simulink model "QD2_MissionCtrl_Swarm_6x_R2021a"  (R2021a)
settings: Solver=ode2  StartTime=0.0  StopTime=inf  FixedStep=0.001  RelTol=1e-3  EnableMultiTasking=on
undefined symbols (not defined in the file): datetime, Host, localhost, m, qc_get_step_size, saved_data
libraries: quarc_library x64, simulink x18, simulink_extras x1
(part 1 of 3)
settings Model: SimulationMode=external  ExtModeTrigDuration=10000  Creator=Admin  LastModifiedBy=jpineros
settings SolverCC: AlgebraicLoopSolver=TrustRegion  PositivePriorityOrder=on
settings DataIOCC: ReturnWorkspaceOutputs=off
settings DebuggingCC: SFUnexpectedBacktrackingDiag=warning  SFNoUnconditionalDefaultTransitionDiag=warning  SFExecutionAtInitializationDiag=none  ArithmeticOperatorsInVariantConditions=warning
settings SFSimCC: SimUseLocalCustomCode=off  CustomCodeUndefinedFunction=UseInterfaceOnly
settings RTWCC: Description=QUARC Win64 Target Using Toolchain  SystemTargetFile=quarc_win64.tlc  TemplateMakefile=quarc_default_tmf  RTWUseLocalCustomCode=off  Toolchain=QUARC win64 | nmake (64-bit Windows)  BuildConfiguration=Faster Runs  DLArmComputeVersion=20.02.1
settings CodeAppCC: StateflowObjectComments=on
settings STFCustomTargetCC: ConcurrentExecutionCompliant=on  SystemTargetFile=quarc_win64.tlc
settings GRTTargetCC: TargetLangStandard=C89/C90 (ANSI)  ParMdlRefBuildCompliant=off  CompOptLevelCompliant=off  CombineOutputUpdateFcns=off  MatFileLogging=off  CPPClassGenCompliant=off  GRTInterface=on  ExtMode=on  ExtModeMexFile=quarc_comm  ExtModeMexArgs='-w -d %d -uri %u -URI_Host_V1 tcpip://localhost:18001 -URI_Host_V2 tcpip://localhost:18002 -URI_Host_V3 tcpip://localhost:18003 -URI_Host_V4 tcpip://localhost:18004 -URI_Host_V5 tcpip://localhost:18005 -URI_Host_V6 tcpip://localhost:18006'
settings ConfigComp: CovMetricSettings=dw  CovSaveCumulativeToWorkspaceVar=on  CovSaveSingleToWorkspaceVar=on  CovExternalEMLEnable=off

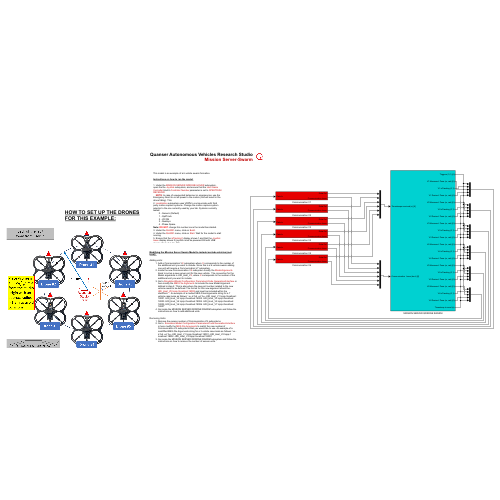
[thumbnail: Simulink's stored preview of the top-level diagram]
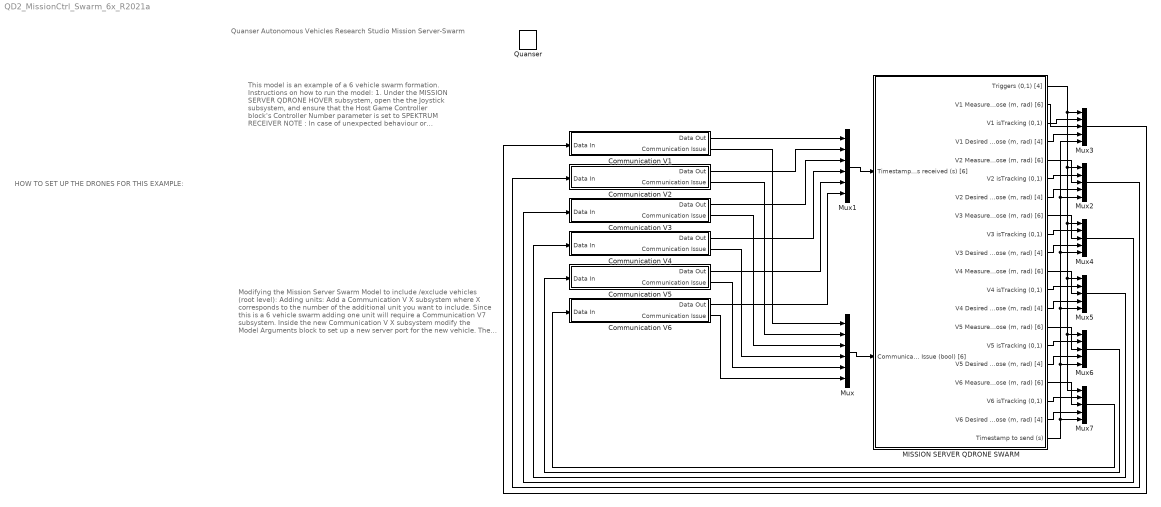
== system QD2_MissionCtrl_Swarm_6x_R2021a ==
  note: Modifying the Mission Server Swarm Model to include /exclude vehicles (root level):
      |
      | Adding units:
      | Add a Communication V X subsystem where X corresponds to the number of the additional unit you want to include. Since this is a 6 vehicle swarm adding one unit will require a Communication V7 subsystem.
      | Inside the new Communication V X subsystem modify the Model Arguments block to set up a new server port for the new vehicle. The convention for the Model arguments is URI_Host_V X , where X corresponds to the number of the additional unit you want to include.
      | Go to Simulation\Model Configuration Parameters\Code Generation\Interface in here modify the MEX-File Arguments to include the new Model Argument defined in step 2. This is also where the new port number related to the new vehicle needs to be defined. The format for this new argument should be -URI_Host_VX tcpip://localhost:1800X and must be included within the identifiers ' ' . An example of a modied MEX-Files Arguments string for a 7 vehicle case looks as follows: '-w -d %d -uri %u -URI_Host_V1 tcpip://localhost:18001 -URI_Host_V2 tcpip://localhost:18002 -URI_Host_V3 tcpip://localhost:18003 -URI_Host_V4 tcpip://localhost:18004 -URI_Host_V5 tcpip://localhost:18005 -URI_Host_V6 tcpip://localhost:18006 -URI_Host_V7 tcpip://localhost:18007'
      | Go inside the MISSION SERVER QDRONE SWARM subsystem and follow the instructions on how to add additional units.
      |
      | Removing Units:
      | Remove the excess number of Communication VX subsystems.
      | Go to Simulation\Model Configuration Parameters\Code Generation\Interface in here modify the MEX-File Arguments to match the new number of Communication VX subsystems that you would like to use. An example of a modifified MEX-File Arguments string for a 3 vehicle case looks as follows: '-w -d %d -uri %u -URI_Host_V1 tcpip://localhost:18001 -URI_Host_V2 tcpip://localhost:18002 -URI_Host_V3 tcpip://localhost:18003'
      | Go inside the MISSION SERVER QDRONE SWARM subsystem and follow the instructions on how to remove the number of excess units.
  note: This model is an example of a 6 vehicle swarm formation.
      |
      | Instructions on how to run the model:
      |
      | 1. Under the MISSION SERVER QDRONE HOVER subsystem, open the the Joystick subsystem, and ensure that the Host Game Controller block's Controller Number parameter is set to SPEKTRUM RECEIVER
      | NOTE : In case of unexpected behaviour or emergencies, use the Emergency Abort to cut all power to the motors (this will result in the drone falling). This
      | 2. Localization subsystem uses VRPN to communicate with third party motion capture systems. Change the motion capture system selector to the one currently used by your lab. Systems currently tested:
      | 0 - Generic (Default)
      | 1 - OptiTrack
      | 2 - VICON
      | 3 - Qualisys
      | 4 - Phase Space
      | Note: DO NOT change this number once the model has started.
      | 3. Under the QUARC menu, click on Build .
      | 4. Under the QUARC menu, click on Start . Wait for the model to start running.
      | 5. Ensure that the isTracking? display shows 1 and that the Joystick Issue display shows 0 (joystick must be powered ON with USB dongle attached to the PC).
      |
      | NOTE : At the start of the model the Comm Issue with Commander display SHOULD display 0. Once the Commander_Stabilizer has successfully connected to the mission server the communication issue flag will update. Landing the QDrones will stop the Commander_Stabilizer model at which point the Comm Issue with Commander should show 1. To close the warning window please stop the Mission_Server_Swarm model.
  note: Quanser Autonomous Vehicles Research Studio
      | Mission Server-Swarm
  note: HOW TO SET UP THE DRONES FOR THIS EXAMPLE:
  Communication V1 : Subsystem
  Communication V2 : Subsystem
  Communication V3 : Subsystem
  Communication V4 : Subsystem
  Communication V5 : Subsystem
  Communication V6 : Subsystem
  MISSION SERVER QDRONE SWARM : Subsystem
  Mux : Mux  Inputs=6
  Mux1 : Mux  Inputs=6
  Mux{2..7} (6 alike) : Mux  Inputs=5
  Quanser : quarc_library/Logos/Quanser
  wires:
  Mux/1 -> MISSION SERVER QDRONE SWARM/2(Communication Issue (bool) [6])
  Mux1/1 -> MISSION SERVER QDRONE SWARM/1(Timestamps received (s) [6])
  MISSION SERVER QDRONE SWARM/3(V1 isTracking (0,1)) -> Mux3/2
  MISSION SERVER QDRONE SWARM/6(V2 isTracking (0,1)) -> Mux2/2
  MISSION SERVER QDRONE SWARM/9(V3 isTracking (0,1)) -> Mux4/2
  MISSION SERVER QDRONE SWARM/12(V4 isTracking (0,1)) -> Mux5/2
  MISSION SERVER QDRONE SWARM/15(V5 isTracking (0,1)) -> Mux6/2
  MISSION SERVER QDRONE SWARM/18(V6 isTracking (0,1)) -> Mux7/2
  MISSION SERVER QDRONE SWARM/1(Triggers (0,1) [4]) -> Mux3/1, Mux2/1, Mux4/1, Mux5/1, Mux6/1, Mux7/1
  MISSION SERVER QDRONE SWARM/4("V1 Desired Pose (m, rad) [4]") -> Mux3/4
  MISSION SERVER QDRONE SWARM/7("V2 Desired Pose (m, rad) [4]") -> Mux2/4
  MISSION SERVER QDRONE SWARM/10("V3 Desired Pose (m, rad) [4]") -> Mux4/4
  MISSION SERVER QDRONE SWARM/13("V4 Desired Pose (m, rad) [4]") -> Mux5/4
  MISSION SERVER QDRONE SWARM/16("V5 Desired Pose (m, rad) [4]") -> Mux6/4
  MISSION SERVER QDRONE SWARM/19("V6 Desired Pose (m, rad) [4]") -> Mux7/4
  MISSION SERVER QDRONE SWARM/20(Timestamp to send (s)) -> Mux3/5, Mux2/5, Mux4/5, Mux5/5, Mux6/5, Mux7/5
  Mux3/1 -> Communication V1/1(Data In)
  Mux2/1 -> Communication V2/1(Data In)
  Mux4/1 -> Communication V3/1(Data In)
  Mux5/1 -> Communication V4/1(Data In)
  Mux6/1 -> Communication V5/1(Data In)
  Mux7/1 -> Communication V6/1(Data In)
  MISSION SERVER QDRONE SWARM/17("V6 Measured Pose (m, rad) [6]") -> Mux7/3
  MISSION SERVER QDRONE SWARM/14("V5 Measured Pose (m, rad) [6]") -> Mux6/3
  MISSION SERVER QDRONE SWARM/11("V4 Measured Pose (m, rad) [6]") -> Mux5/3
  MISSION SERVER QDRONE SWARM/8("V3 Measured  Pose (m, rad) [6]") -> Mux4/3
  MISSION SERVER QDRONE SWARM/5("V2 Measured Pose (m, rad) [6]") -> Mux2/3
  MISSION SERVER QDRONE SWARM/2("V1 Measured Pose (m, rad) [6]") -> Mux3/3
  Communication V1/1(Data Out) -> Mux1/1
  Communication V2/1(Data Out) -> Mux1/2
  Communication V3/1(Data Out) -> Mux1/3
  Communication V4/1(Data Out) -> Mux1/4
  Communication V5/1(Data Out) -> Mux1/5
  Communication V6/1(Data Out) -> Mux1/6
  Communication V1/2(Communication Issue) -> Mux/1
  Communication V2/2(Communication Issue) -> Mux/2
  Communication V3/2(Communication Issue) -> Mux/3
  Communication V4/2(Communication Issue) -> Mux/4
  Communication V5/2(Communication Issue) -> Mux/5
  Communication V6/2(Communication Issue) -> Mux/6

== system QD2_MissionCtrl_Swarm_6x_R2021a/Communication V1 ==
  Data In : Inport
  Constant : Constant
  Detect Communication loss : Subsystem
  Model Argument : quarc_library/Sources/Signals/Model Argument  argument_name=URI_Host_V1  has_value=on  data_type_mode=Specify via dialog  data_type=char  max_length=80  default_value=0  default_string=tcpip://localhost:18001  variable_size=off
      settings: AttributesFormatString=(-%<argument_name>)  SourceProductName=QUARC Targets
  Stream Server : quarc_library/Communications/Basic/Stream Server  uri_source=External input port  uri=tcpip://localhost:18877  send_buffer_size=1460  receive_buffer_size=1460  byte_order=little endian (Intel - LSB first)  optimization=Minimum latency  send_options=Send most recent data  receive_options=Receive most recent data  default_value=zeros(1,1)  sample_time=qc_get_step_size  active=off  implementation=Use blocking I/O in a separate thread  send_fifo_size=1000  receive_fifo_size=1000  send_priority=0  receive_priority=0  send_dimensions=off  receive_dimensions=off  max_dimensions=-1  data_type=Inherited via back propagation  type_expr=BusObject
  "String Display " : quarc_library/Strings/String Display  alignment=center  display_mode=Single line  sample_time=-1  use_new=off
      settings: SourceProductName=QUARC Targets
  Terminator1 : Terminator
  Terminator2 : Terminator
  Data Out : Outport  VectorParamsAs1DForOutWhenUnconnected=off
  Communication Issue : Outport  Port=2  VectorParamsAs1DForOutWhenUnconnected=off
  wires:
  Detect Communication loss/1(Communication Issue (0,1)) -> Communication Issue/1
  Stream Server/1 -> Detect Communication loss/1(State)
  Stream Server/2 -> Detect Communication loss/2(Error)
  Stream Server/4 -> Data Out/1
  Model Argument/1 -> Stream Server/3, "String Display "/1
  Stream Server/5 -> Terminator1/1
  Stream Server/3 -> Terminator2/1
  Data In/1 -> Stream Server/1
  Constant/1 -> Stream Server/2

== system QD2_MissionCtrl_Swarm_6x_R2021a/Communication V2 ==
  Data In : Inport
  Constant : Constant
  Detect Communication loss : Subsystem
  Model Argument : quarc_library/Sources/Signals/Model Argument  argument_name=URI_Host_V2  has_value=on  data_type_mode=Specify via dialog  data_type=char  max_length=80  default_value=0  default_string=tcpip://localhost:18002  variable_size=off
      settings: AttributesFormatString=(-%<argument_name>)  SourceProductName=QUARC Targets
  Stream Server : quarc_library/Communications/Basic/Stream Server  uri_source=External input port  uri=tcpip://localhost:18877  send_buffer_size=1460  receive_buffer_size=1460  byte_order=little endian (Intel - LSB first)  optimization=Minimum latency  send_options=Send most recent data  receive_options=Receive most recent data  default_value=zeros(1,1)  sample_time=qc_get_step_size  active=off  implementation=Use blocking I/O in a separate thread  send_fifo_size=1000  receive_fifo_size=1000  send_priority=0  receive_priority=0  send_dimensions=off  receive_dimensions=off  max_dimensions=-1  data_type=Inherited via back propagation  type_expr=BusObject
  "String Display " : quarc_library/Strings/String Display  alignment=center  display_mode=Single line  sample_time=-1  use_new=off
      settings: SourceProductName=QUARC Targets
  Terminator1 : Terminator
  Terminator2 : Terminator
  Data Out : Outport  VectorParamsAs1DForOutWhenUnconnected=off
  Communication Issue : Outport  Port=2  VectorParamsAs1DForOutWhenUnconnected=off
  wires:
  Constant/1 -> Stream Server/2
  Data In/1 -> Stream Server/1
  Stream Server/3 -> Terminator2/1
  Stream Server/5 -> Terminator1/1
  Model Argument/1 -> "String Display "/1, Stream Server/3
  Stream Server/4 -> Data Out/1
  Stream Server/2 -> Detect Communication loss/2(Error)
  Stream Server/1 -> Detect Communication loss/1(State)
  Detect Communication loss/1(Communication Issue (0,1)) -> Communication Issue/1

== system QD2_MissionCtrl_Swarm_6x_R2021a/Communication V3 ==
  Data In : Inport
  Constant : Constant
  Detect Communication loss : Subsystem
  Model Argument : quarc_library/Sources/Signals/Model Argument  argument_name=URI_Host_V3  has_value=on  data_type_mode=Specify via dialog  data_type=char  max_length=80  default_value=0  default_string=tcpip://localhost:18003  variable_size=off
      settings: AttributesFormatString=(-%<argument_name>)  SourceProductName=QUARC Targets
  Stream Server : quarc_library/Communications/Basic/Stream Server  uri_source=External input port  uri=tcpip://localhost:18877  send_buffer_size=1460  receive_buffer_size=1460  byte_order=little endian (Intel - LSB first)  optimization=Minimum latency  send_options=Send most recent data  receive_options=Receive most recent data  default_value=zeros(1,1)  sample_time=qc_get_step_size  active=off  implementation=Use blocking I/O in a separate thread  send_fifo_size=1000  receive_fifo_size=1000  send_priority=0  receive_priority=0  send_dimensions=off  receive_dimensions=off  max_dimensions=-1  data_type=Inherited via back propagation  type_expr=BusObject
  "String Display " : quarc_library/Strings/String Display  alignment=center  display_mode=Single line  sample_time=-1  use_new=off
      settings: SourceProductName=QUARC Targets
  Terminator1 : Terminator
  Terminator2 : Terminator
  Data Out : Outport  VectorParamsAs1DForOutWhenUnconnected=off
  Communication Issue : Outport  Port=2  VectorParamsAs1DForOutWhenUnconnected=off
  wires:
  Detect Communication loss/1(Communication Issue (0,1)) -> Communication Issue/1
  Stream Server/1 -> Detect Communication loss/1(State)
  Stream Server/2 -> Detect Communication loss/2(Error)
  Stream Server/4 -> Data Out/1
  Model Argument/1 -> Stream Server/3, "String Display "/1
  Stream Server/5 -> Terminator1/1
  Stream Server/3 -> Terminator2/1
  Data In/1 -> Stream Server/1
  Constant/1 -> Stream Server/2

== system QD2_MissionCtrl_Swarm_6x_R2021a/Communication V4 ==
  Data In : Inport
  Constant : Constant
  Detect Communication loss : Subsystem
  Model Argument : quarc_library/Sources/Signals/Model Argument  argument_name=URI_Host_V4  has_value=on  data_type_mode=Specify via dialog  data_type=char  max_length=80  default_value=0  default_string=tcpip://localhost:18004  variable_size=off
      settings: AttributesFormatString=(-%<argument_name>)  SourceProductName=QUARC Targets
  Stream Server : quarc_library/Communications/Basic/Stream Server  uri_source=External input port  uri=tcpip://localhost:18877  send_buffer_size=1460  receive_buffer_size=1460  byte_order=little endian (Intel - LSB first)  optimization=Minimum latency  send_options=Send most recent data  receive_options=Receive most recent data  default_value=zeros(1,1)  sample_time=qc_get_step_size  active=off  implementation=Use blocking I/O in a separate thread  send_fifo_size=1000  receive_fifo_size=1000  send_priority=0  receive_priority=0  send_dimensions=off  receive_dimensions=off  max_dimensions=-1  data_type=Inherited via back propagation  type_expr=BusObject
  "String Display " : quarc_library/Strings/String Display  alignment=center  display_mode=Single line  sample_time=-1  use_new=off
      settings: SourceProductName=QUARC Targets
  Terminator1 : Terminator
  Terminator2 : Terminator
  Data Out : Outport  VectorParamsAs1DForOutWhenUnconnected=off
  Communication Issue : Outport  Port=2  VectorParamsAs1DForOutWhenUnconnected=off
  wires:
  Constant/1 -> Stream Server/2
  Data In/1 -> Stream Server/1
  Stream Server/3 -> Terminator2/1
  Stream Server/5 -> Terminator1/1
  Model Argument/1 -> "String Display "/1, Stream Server/3
  Stream Server/4 -> Data Out/1
  Stream Server/2 -> Detect Communication loss/2(Error)
  Stream Server/1 -> Detect Communication loss/1(State)
  Detect Communication loss/1(Communication Issue (0,1)) -> Communication Issue/1

== system QD2_MissionCtrl_Swarm_6x_R2021a/Communication V5 ==
  Data In : Inport
  Constant : Constant
  Detect Communication loss : Subsystem
  Model Argument : quarc_library/Sources/Signals/Model Argument  argument_name=URI_Host_V5  has_value=on  data_type_mode=Specify via dialog  data_type=char  max_length=80  default_value=0  default_string=tcpip://localhost:18005  variable_size=off
      settings: AttributesFormatString=(-%<argument_name>)  SourceProductName=QUARC Targets
  Stream Server : quarc_library/Communications/Basic/Stream Server  uri_source=External input port  uri=tcpip://localhost:18877  send_buffer_size=1460  receive_buffer_size=1460  byte_order=little endian (Intel - LSB first)  optimization=Minimum latency  send_options=Send most recent data  receive_options=Receive most recent data  default_value=zeros(1,1)  sample_time=qc_get_step_size  active=off  implementation=Use blocking I/O in a separate thread  send_fifo_size=1000  receive_fifo_size=1000  send_priority=0  receive_priority=0  send_dimensions=off  receive_dimensions=off  max_dimensions=-1  data_type=Inherited via back propagation  type_expr=BusObject
  "String Display " : quarc_library/Strings/String Display  alignment=center  display_mode=Single line  sample_time=-1  use_new=off
      settings: SourceProductName=QUARC Targets
  Terminator1 : Terminator
  Terminator2 : Terminator
  Data Out : Outport  VectorParamsAs1DForOutWhenUnconnected=off
  Communication Issue : Outport  Port=2  VectorParamsAs1DForOutWhenUnconnected=off
  wires:
  Detect Communication loss/1(Communication Issue (0,1)) -> Communication Issue/1
  Stream Server/1 -> Detect Communication loss/1(State)
  Stream Server/2 -> Detect Communication loss/2(Error)
  Stream Server/4 -> Data Out/1
  Model Argument/1 -> Stream Server/3, "String Display "/1
  Stream Server/5 -> Terminator1/1
  Stream Server/3 -> Terminator2/1
  Data In/1 -> Stream Server/1
  Constant/1 -> Stream Server/2

== system QD2_MissionCtrl_Swarm_6x_R2021a/Communication V6 ==
  Data In : Inport
  Constant : Constant
  Detect Communication loss : Subsystem
  Model Argument : quarc_library/Sources/Signals/Model Argument  argument_name=URI_Host_V6  has_value=on  data_type_mode=Specify via dialog  data_type=char  max_length=80  default_value=0  default_string=tcpip://localhost:18006  variable_size=off
      settings: AttributesFormatString=(-%<argument_name>)  SourceProductName=QUARC Targets
  Stream Server : quarc_library/Communications/Basic/Stream Server  uri_source=External input port  uri=tcpip://localhost:18877  send_buffer_size=1460  receive_buffer_size=1460  byte_order=little endian (Intel - LSB first)  optimization=Minimum latency  send_options=Send most recent data  receive_options=Receive most recent data  default_value=zeros(1,1)  sample_time=qc_get_step_size  active=off  implementation=Use blocking I/O in a separate thread  send_fifo_size=1000  receive_fifo_size=1000  send_priority=0  receive_priority=0  send_dimensions=off  receive_dimensions=off  max_dimensions=-1  data_type=Inherited via back propagation  type_expr=BusObject
  "String Display " : quarc_library/Strings/String Display  alignment=center  display_mode=Single line  sample_time=-1  use_new=off
      settings: SourceProductName=QUARC Targets
  Terminator1 : Terminator
  Terminator2 : Terminator
  Data Out : Outport  VectorParamsAs1DForOutWhenUnconnected=off
  Communication Issue : Outport  Port=2  VectorParamsAs1DForOutWhenUnconnected=off
  wires:
  Constant/1 -> Stream Server/2
  Data In/1 -> Stream Server/1
  Stream Server/3 -> Terminator2/1
  Stream Server/5 -> Terminator1/1
  Model Argument/1 -> "String Display "/1, Stream Server/3
  Stream Server/4 -> Data Out/1
  Stream Server/2 -> Detect Communication loss/2(Error)
  Stream Server/1 -> Detect Communication loss/1(State)
  Detect Communication loss/1(Communication Issue (0,1)) -> Communication Issue/1

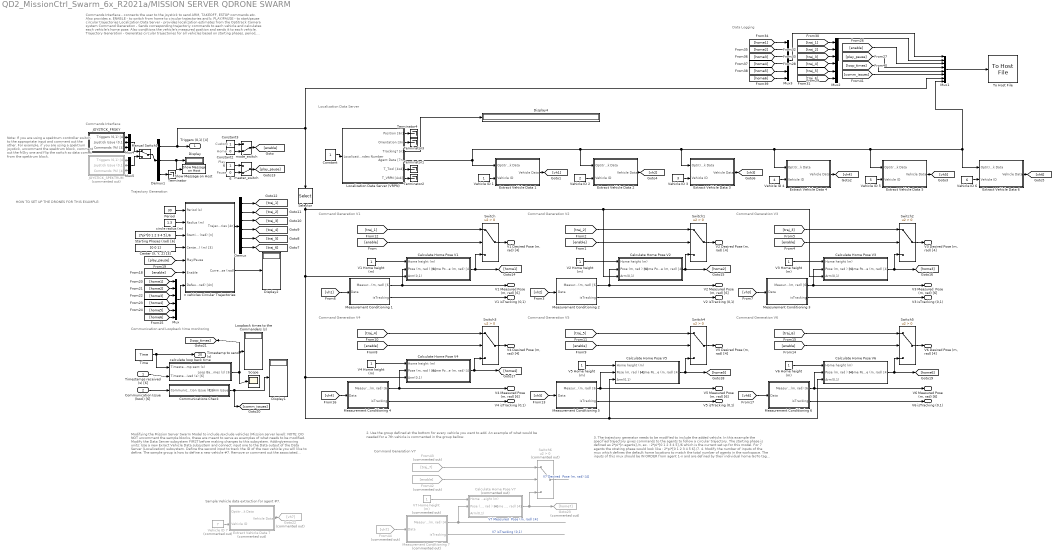
== system QD2_MissionCtrl_Swarm_6x_R2021a/MISSION SERVER QDRONE SWARM ==
  note: 3. The trajectory generator needs to be modified to include the added vehicle. In this example
      | the specified trajectory gives commands to the agents to follow a circular trajectory. The starting phase
      | is defined as 2*pi*[n agents]./n, ex. : 2*pi*[0 1 2 3 4 5]./6 which is the current set up for this model. For
      | 7 agents the strating phase would look like : 2*pi*[0 1 2 3 4 5 6]./7.
      |
      | 4. Modify the number of inputs of the mux which defines the default home locations to match the
      | total number of agents in the workspace. The inputs of this mux should be IN ORDER from agent 1-n and
      | are defined by their individual home GoTo tag as seen in the default group commented out in step 7.
      |
      | 5. Adjust the communication and loopback time monitoring logic to add or remove associated
      | sub-blocks as needed.
  note: 2. Use the group defined at the bottom for every vehicle you want to add. An example of what would be needed for a 7th vehicle is commented in the group bellow.
  note: Sample Vehicle data extraction for agent #7.
  note: Modifying the Mission Server Swarm Model to include /exclude vehicles (Mission server level):
      |
      | NOTE: DO NOT uncomment the sample blocks, these are meant to serve as examples of what needs to be modified. Modify the Data Server subsystem FIRST before making changes to this subsystem.
      |
      | Adding\removing units:
      | Use a new Exract Vehicle Data subsystem and connect input one to the Data output of the Data Server (Localization) subsystem. Define the second input to track the ID of the new vehicle you will like to define. The sample group is how to define a new vehicle #7.
      | Remove or comment out the associated subsystem blocks for less number of vehicles.
  note: Commands Interface - connects the user to the joystick to send ARM, TAKEOFF, ESTOP commands etc. Also provides a. ENABLE - to switch from home to circular trajectories and b. PLAY/PAUSE - to start/pause circular trajectories
      | Localization Data Server - provides localization estimates from the Optitrack Camera system
      | Command Generation - Sends corresponding trajectoriy commands to each vehicle and calculates each vehicle's home pose. Also conditions the vehicle's measured position and sends it to each vehicle.
      | Trajectory Generation - Generates circular trajectories for all vehicles based on starting phases, period, radus and center location. When ENABLE is low, it switches to the trajectory at the Default (m, rad) [4] input
      | Communication and Loopback time monitoring - monitors communication issues with any vehicle, and also displays the loopback time to each model (time taken to send a packet to a vehicle and receive it back immediately).
  note: Data Logging
  note: Communication and Loopback time monitoring
  note: Trajectory Generation
  note: Localization Data Server
  note: Commands Interface
  note: Home
  note: Custom
  note: Command Generation V1
  note: Command Generation V2
  note: Command Generation V3
  note: Command Generation V4
  note: Command Generation V5
  note: Command Generation V6
  note: Pause
  note: Play
  note: Command Generation V7
  note: HOW TO SET UP THE DRONES FOR THIS EXAMPLE:
  note: Note:
      | If you are using a spektrum controller switch to the appropriate input and comment out the other.
      | For example, if you are using a spektrum joystick, uncomment the spektrum block, comment out the frSky one and flip the switch so data comes from the spektrum block.
  Timestamps received (s) [6] : Inport
  Communication Issue (bool) [6] : Inport  Port=2
  "          6" : Constant
  "   6" : Constant  Value=0
  Calculate Home Pose V1 : Subsystem
  Calculate Home Pose V2 : Subsystem
  Calculate Home Pose V3 : Subsystem
  Calculate Home Pose V4 : Subsystem
  Calculate Home Pose V5 : Subsystem
  Calculate Home Pose V6 : Subsystem
  Calculate Home Pose V7 : Subsystem  Commented=on
  "Center (X, Y, Z) [3]" : Constant  Value=[0 0 1]
  Communications Check : Subsystem
  Constant : Constant
  Constant2 : Constant  Value=0
  Constant3 : Constant
  Demux : Demux  Outputs=[4 4 4 4 4 4]
  Demux1 : Demux  Outputs=[4 1 4]
  Display{,1..2,4} (4 alike) : Display
  Extract Vehicle Data 1 : Subsystem
  Extract Vehicle Data 2 : Subsystem
  Extract Vehicle Data 3 : Subsystem
  Extract Vehicle Data 4 : Subsystem
  Extract Vehicle Data 5 : Subsystem
  Extract Vehicle Data 6 : Subsystem
  Extract Vehicle Data 7 : Subsystem  Commented=on
  From42 : From  Commented=on  GotoTag=enable
  From43 : From  Commented=on  GotoTag=traj_7
  From44 : From  Commented=on  GotoTag=vh7
  Goto22 : Goto  Commented=on  GotoTag=vh7
  Goto23 : Goto  Commented=on  GotoTag=home7
  JOYSTICK_FRSKY : Subsystem
      mask Display: image('$imagefile'); % Use "Edit Image" on toolstrip to change.
  JOYSTICK_SPEKTRUM : Subsystem  Commented=on
      mask Display: image('$imagefile'); % Use "Edit Image" on toolstrip to change.
  "Localization Data Server (VRPN) " : Subsystem
  Loopback times to the Commanders (s) : Display
  Manual Switch1 : ManualSwitch
  Measurement Conditioning 1 : Subsystem
  Measurement Conditioning 2 : Subsystem
  Measurement Conditioning 3 : Subsystem
  Measurement Conditioning 4 : Subsystem
  Measurement Conditioning 5 : Subsystem
  Measurement Conditioning 6 : Subsystem
  Measurement Conditioning 7 : Subsystem  Commented=on
  Mux : Mux  Inputs=6
  Mux1 : Mux  Inputs=8
  Mux2 : Mux  Inputs=6
  Mux3 : Mux  Inputs=6
  Mux4 : Mux  Inputs=[4 1 4]
  Mux5 : Mux  Inputs=[4 1 4]
  Period : Constant  Value=30
  Scope : Scope
  Selector : Selector  InputPortWidth=4  IndexOptions=Index vector (dialog)  Indices=[1]  OutputSizes=1
  "Show Message on Host " : quarc_library/Sinks/Error Handling/Show Message on Host  message_type=Fixed error message  message_icon=Warning  message=Mission Server: Joystick Disconnected
      settings: AttributesFormatString="\"%<message>\""  SourceProductName=QUARC Targets
  Starting Phases (rad) [6] : Constant  Value=2*pi*[0 1 2 3 4 5]./6
  Switch{,1..5} (6 alike) : Switch  Criteria=u2 > Threshold
  Switch6 : Switch  Commented=on  Criteria=u2 > Threshold
  Terminator{,1..4} (5 alike) : Terminator
  Time : quarc_library/Sources/Time/Time  time_source=Wall clock  sample_time=qc_get_step_size
  To Host File : quarc_library/Sinks/To Host/To Host File  source=Specify via dialog (do not evaluate)  file_name=saved_data/%m/%{char(datetime)}.mat  variable_name=data  decimation=1  sample_time=-1  file_format=MAT-file v.4  options=No header or footer  append=off  final_file_name=saved_data/QD2_MissionCtrl_Swarm_6x_R2021a_/2025-02-21 15-27-59.mat  bitrate=2000000
  V1 Home height (m) : Constant
  V2 Home height (m) : Constant
  V3 Home height (m) : Constant
  V4 Home height (m) : Constant
  V5 Home height (m) : Constant
  V6 Home height (m) : Constant
  V7 Home height (m) : Constant  Commented=on
  Vehicle ID 1 : Constant
  "Vehicle ID 2 " : Constant  Value=2
  Vehicle ID 3 : Constant  Value=3
  Vehicle ID 4 : Constant  Value=4
  Vehicle ID 5 : Constant  Value=5
  Vehicle ID 6 : Constant  Value=6
  Vehicle ID 7 : Constant  Commented=on  Value=7
  calculate loop back time : Subsystem
  circle radius (m) : Constant  Value=1.3
  master_switch : ManualSwitch  CurrentSetting=0
  mode_switch : ManualSwitch  CurrentSetting=0
  n vehicles Circular Trajectories : Subsystem
  Triggers (0,1) [4] : Outport  VectorParamsAs1DForOutWhenUnconnected=off
  "V1 Measured Pose (m, rad) [6]" : Outport  Port=2  VectorParamsAs1DForOutWhenUnconnected=off
  V1 isTracking (0,1) : Outport  Port=3  VectorParamsAs1DForOutWhenUnconnected=off
  "V1 Desired Pose (m, rad) [4]" : Outport  Port=4  VectorParamsAs1DForOutWhenUnconnected=off
  "V2 Measured Pose (m, rad) [6]" : Outport  Port=5  VectorParamsAs1DForOutWhenUnconnected=off
  V2 isTracking (0,1) : Outport  Port=6  VectorParamsAs1DForOutWhenUnconnected=off
  "V2 Desired Pose (m, rad) [4]" : Outport  Port=7  VectorParamsAs1DForOutWhenUnconnected=off
  "V3 Measured  Pose (m, rad) [6]" : Outport  Port=8  VectorParamsAs1DForOutWhenUnconnected=off
  V3 isTracking (0,1) : Outport  Port=9  VectorParamsAs1DForOutWhenUnconnected=off
  "V3 Desired Pose (m, rad) [4]" : Outport  Port=10  VectorParamsAs1DForOutWhenUnconnected=off
  "V4 Measured Pose (m, rad) [6]" : Outport  Port=11  VectorParamsAs1DForOutWhenUnconnected=off
  V4 isTracking (0,1) : Outport  Port=12  VectorParamsAs1DForOutWhenUnconnected=off
  "V4 Desired Pose (m, rad) [4]" : Outport  Port=13  VectorParamsAs1DForOutWhenUnconnected=off
  "V5 Measured Pose (m, rad) [6]" : Outport  Port=14  VectorParamsAs1DForOutWhenUnconnected=off
  V5 isTracking (0,1) : Outport  Port=15  VectorParamsAs1DForOutWhenUnconnected=off
  "V5 Desired Pose (m, rad) [4]" : Outport  Port=16  VectorParamsAs1DForOutWhenUnconnected=off
  "V6 Measured Pose (m, rad) [6]" : Outport  Port=17  VectorParamsAs1DForOutWhenUnconnected=off
  V6 isTracking (0,1) : Outport  Port=18  VectorParamsAs1DForOutWhenUnconnected=off
  "V6 Desired Pose (m, rad) [4]" : Outport  Port=19  VectorParamsAs1DForOutWhenUnconnected=off
  Timestamp to send (s) : Outport  Port=20  VectorParamsAs1DForOutWhenUnconnected=off
  wires:
  Demux1/2 -> Display/1, "Show Message on Host "/1
  Constant3/1 -> mode_switch/1
  Constant2/1 -> mode_switch/2
  Demux1/3 -> Terminator/1
  "   6"/1 -> master_switch/2
  Period/1 -> n vehicles Circular Trajectories/1(Period (s))
  circle radius (m)/1 -> n vehicles Circular Trajectories/2(Radius (m))
  "          6"/1 -> master_switch/1
  [play_pause] -> n vehicles Circular Trajectories/5(Play/Pause)
  Demux1/1 -> Triggers (0,1) [4]/1, Mux1/7, Selector/1
  Time/1 -> Timestamp to send (s)/1, calculate loop back time/1(Timestamp sent (s))
  Timestamps received (s) [6]/1 -> calculate loop back time/2(Timestamps received (s) [6])
  Starting Phases (rad) [6]/1 -> n vehicles Circular Trajectories/3(Starting Phase (rad) [n])
  "Center (X, Y, Z) [3]"/1 -> n vehicles Circular Trajectories/4(Center (X,Y,Z) (m) [3])
  n vehicles Circular Trajectories/2(Current Phase (rad)) -> Display2/1
  Vehicle ID 6/1 -> Extract Vehicle Data 6/2(Vehicle ID)
  Vehicle ID 5/1 -> Extract Vehicle Data 5/2(Vehicle ID)
  Vehicle ID 3/1 -> Extract Vehicle Data 3/2(Vehicle ID)
  "Vehicle ID 2 "/1 -> Extract Vehicle Data 2/2(Vehicle ID)
  "Localization Data Server (VRPN) "/4(Agent Data [7n]) -> Extract Vehicle Data 2/1(Optitrack Data), Extract Vehicle Data 3/1(Optitrack Data), Extract Vehicle Data 4/1(Optitrack Data), Extract Vehicle Data 5/1(Optitrack Data), Mux1/8, Extract Vehicle Data 6/1(Optitrack Data), Extract Vehicle Data 1/1(Optitrack Data)
  Vehicle ID 1/1 -> Extract Vehicle Data 1/2(Vehicle ID)
  Vehicle ID 4/1 -> Extract Vehicle Data 4/2(Vehicle ID)
  Measurement Conditioning 1/2(isTracking) -> V1 isTracking (0,1)/1
  Calculate Home Pose V1/1("Home Pose (m, rad) [4]") -> [home1], Switch/3
  [traj_1] -> Switch/1
  V1 Home height (m)/1 -> Calculate Home Pose V1/1(Home height (m))
  Measurement Conditioning 1/1("Measured Pose (m, rad) [6]") -> Calculate Home Pose V1/2("Pose (m, rad ) [4]"), "V1 Measured Pose (m, rad) [6]"/1
  Switch/1 -> "V1 Desired Pose (m, rad) [4]"/1
  mode_switch/1 -> [enable]
  [enable] -> Switch/2
  Extract Vehicle Data 1/1(Vehicle Data) -> [vh1]
  Extract Vehicle Data 4/1(Vehicle Data) -> [vh4]
  Extract Vehicle Data 5/1(Vehicle Data) -> [vh5]
  Extract Vehicle Data 2/1(Vehicle Data) -> [vh2]
  Extract Vehicle Data 6/1(Vehicle Data) -> [vh6]
  Extract Vehicle Data 3/1(Vehicle Data) -> [vh3]
  [vh1] -> Measurement Conditioning 1/1(Data)
  n vehicles Circular Trajectories/1(Trajectories [4n]) -> Demux/1
  Demux/1 -> [traj_1]
  Demux/2 -> [traj_2]
  Demux/3 -> [traj_3]
  Demux/4 -> [traj_4]
  Demux/5 -> [traj_5]
  Demux/6 -> [traj_6]
  [vh2] -> Measurement Conditioning 2/1(Data)
  [enable] -> Switch1/2
  Switch1/1 -> "V2 Desired Pose (m, rad) [4]"/1
  Measurement Conditioning 2/1("Measured Pose (m, rad) [6]") -> Calculate Home Pose V2/2("Pose (m, rad ) [4]"), "V2 Measured Pose (m, rad) [6]"/1
  V2 Home height (m)/1 -> Calculate Home Pose V2/1(Home height (m))
  [traj_2] -> Switch1/1
  Calculate Home Pose V2/1("Home Pose (m, rad) [4]") -> [home2], Switch1/3
  Measurement Conditioning 2/2(isTracking) -> V2 isTracking (0,1)/1
  Measurement Conditioning 3/2(isTracking) -> V3 isTracking (0,1)/1
  Calculate Home Pose V3/1("Home Pose (m, rad) [4]") -> [home3], Switch2/3
  [traj_3] -> Switch2/1
  V3 Home height (m)/1 -> Calculate Home Pose V3/1(Home height (m))
  Measurement Conditioning 3/1("Measured Pose (m, rad) [6]") -> "V3 Measured  Pose (m, rad) [6]"/1, Calculate Home Pose V3/2("Pose (m, rad ) [4]")
  Switch2/1 -> "V3 Desired Pose (m, rad) [4]"/1
  [enable] -> Switch2/2
  [vh3] -> Measurement Conditioning 3/1(Data)
  [vh6] -> Measurement Conditioning 6/1(Data)
  [enable] -> Switch5/2
  Switch5/1 -> "V6 Desired Pose (m, rad) [4]"/1
  Measurement Conditioning 6/1("Measured Pose (m, rad) [6]") -> "V6 Measured Pose (m, rad) [6]"/1, Calculate Home Pose V6/2("Pose (m, rad ) [4]")
  V6 Home height (m)/1 -> Calculate Home Pose V6/1(Home height (m))
  [traj_6] -> Switch5/1
  Calculate Home Pose V6/1("Home Pose (m, rad) [4]") -> [home6], Switch5/3
  Measurement Conditioning 6/2(isTracking) -> V6 isTracking (0,1)/1
  Measurement Conditioning 5/2(isTracking) -> V5 isTracking (0,1)/1
  Calculate Home Pose V5/1("Home Pose (m, rad) [4]") -> [home5], Switch4/3
  [traj_5] -> Switch4/1
  V5 Home height (m)/1 -> Calculate Home Pose V5/1(Home height (m))
  Measurement Conditioning 5/1("Measured Pose (m, rad) [6]") -> "V5 Measured Pose (m, rad) [6]"/1, Calculate Home Pose V5/2("Pose (m, rad ) [4]")
  Switch4/1 -> "V5 Desired Pose (m, rad) [4]"/1
  [enable] -> Switch4/2
  [vh5] -> Measurement Conditioning 5/1(Data)
  [vh4] -> Measurement Conditioning 4/1(Data)
  [enable] -> Switch3/2
  Switch3/1 -> "V4 Desired Pose (m, rad) [4]"/1
  Measurement Conditioning 4/1("Measured Pose (m, rad) [6]") -> Calculate Home Pose V4/2("Pose (m, rad ) [4]"), "V4 Measured Pose (m, rad) [6]"/1
  V4 Home height (m)/1 -> Calculate Home Pose V4/1(Home height (m))
  [traj_4] -> Switch3/1
  Calculate Home Pose V4/1("Home Pose (m, rad) [4]") -> [home4], Switch3/3
  Measurement Conditioning 4/2(isTracking) -> V4 isTracking (0,1)/1
  [enable] -> n vehicles Circular Trajectories/6(Enable)
  master_switch/1 -> [play_pause]
  Communication Issue (bool) [6]/1 -> Communications Check/1(Communication Issue (0,1))
  calculate loop back time/1(Loop Back Tmes (s) [6]) -> Scope/1, Loopback times to the Commanders (s)/1, [loop_times]
  Mux/1 -> n vehicles Circular Trajectories/7("Default (m, rad) [4n]")
  [home2] -> Mux/2
  [home3] -> Mux/3
  [home4] -> Mux/4
  [home5] -> Mux/5
  [home6] -> Mux/6
  [home1] -> Mux/1
  Mux1/1 -> To Host File/1
  [play_pause] -> Mux1/4
  [enable] -> Mux1/3
  Mux2/1 -> Mux1/2
  [home1] -> Mux3/1
  [home4] -> Mux3/4
  [home3] -> Mux3/3
  [home2] -> Mux3/2
  [home5] -> Mux3/5
  [home6] -> Mux3/6
  [traj_6] -> Mux2/6
  [traj_5] -> Mux2/5
  [traj_4] -> Mux2/4
  [traj_3] -> Mux2/3
  [traj_2] -> Mux2/2
  [traj_1] -> Mux2/1
  Mux3/1 -> Mux1/1
  Communications Check/1(Comm Issue) -> Display1/1, [comm_issues]
  [comm_issues] -> Mux1/6
  [loop_times] -> Mux1/5
  Extract Vehicle Data 7/1(Vehicle Data) -> Goto22/1
  Vehicle ID 7/1 -> Extract Vehicle Data 7/2(Vehicle ID)
  From42/1 -> Switch6/2
  Switch6/1 -> ?  "V7 Desired  Pose (m, rad) [4]"
  From44/1 -> Measurement Conditioning 7/1(Data)
  Measurement Conditioning 7/2(isTracking) -> ?  "V7 isTracking (0,1)"
  From43/1 -> Switch6/1
  V7 Home height (m)/1 -> Calculate Home Pose V7/1(Home height (m))
  Calculate Home Pose V7/1("Home Pose (m, rad) [4]") -> Goto23/1, Switch6/3
  Measurement Conditioning 7/1("Measured Pose (m, rad) [4]") -> Calculate Home Pose V7/2("Pose (m, rad ) [4]")  "V7 Measured  Pose (m, rad) [4]"
  Selector/1 -> Calculate Home Pose V1/3(Arm(0,1)), Calculate Home Pose V6/3(Arm(0,1)), Calculate Home Pose V5/3(Arm(0,1)), Calculate Home Pose V4/3(Arm(0,1)), Calculate Home Pose V3/3(Arm(0,1)), Calculate Home Pose V2/3(Arm(0,1))
  ? -> Calculate Home Pose V7/3(Arm(0,1))
  Mux5/1 -> Manual Switch1/2
  Manual Switch1/1 -> Demux1/1
  JOYSTICK_FRSKY/3(Commands (%) [4]) -> Mux4/3
  JOYSTICK_SPEKTRUM/1(Triggers (0,1) [4]) -> Mux5/1
  JOYSTICK_SPEKTRUM/2(Joystick Issue (0,1)) -> Mux5/2
  JOYSTICK_FRSKY/2(Joystick Issue (0,1)) -> Mux4/2
  JOYSTICK_FRSKY/1(Triggers (0,1) [4]) -> Mux4/1
  JOYSTICK_SPEKTRUM/3(Commands (%) [4]) -> Mux5/3
  Mux4/1 -> Manual Switch1/1
  Constant/1 -> "Localization Data Server (VRPN) "/1(Localization System Index Number)
  "Localization Data Server (VRPN) "/5(T_Tool [4x4]) -> Terminator1/1
  "Localization Data Server (VRPN) "/6(T_VRPN [4x4]) -> Terminator2/1
  "Localization Data Server (VRPN) "/3(Tracking? [n]) -> Display4/1
  "Localization Data Server (VRPN) "/2(Orientation [3n]) -> Terminator3/1
  "Localization Data Server (VRPN) "/1(Position [3n]) -> Terminator4/1

== system QD2_MissionCtrl_Swarm_6x_R2021a/Communication V1/Detect Communication loss ==
  State : Inport
  Error : Inport  Port=2
  Data Type Conversion : DataTypeConversion
  MATLAB Function : MATLAB Function  TreatAsAtomicUnit=on
  Terminator2 : Terminator
  Threshold : quarc_library/Discontinuities/Threshold  operator=>=  param_src=Specify via dialog  threshold=0.5  duration=0.1
      settings: SourceProductName=QUARC Targets
  Time : quarc_library/Sources/Time/Time  time_source=Wall clock  sample_time=qc_get_step_size
  Communication Issue (0,1) : Outport  VectorParamsAs1DForOutWhenUnconnected=off
  wires:
  Threshold/1 -> Data Type Conversion/1
  Data Type Conversion/1 -> Communication Issue (0,1)/1
  Threshold/2 -> Terminator2/1
  Time/1 -> MATLAB Function/1(time)
  State/1 -> MATLAB Function/2(state)
  MATLAB Function/1(stream_connection_loss) -> Threshold/1
  Error/1 -> MATLAB Function/3(error)

== system QD2_MissionCtrl_Swarm_6x_R2021a/Communication V2/Detect Communication loss ==
  State : Inport
  Error : Inport  Port=2
  Data Type Conversion : DataTypeConversion
  MATLAB Function : MATLAB Function  TreatAsAtomicUnit=on
  Terminator2 : Terminator
  Threshold : quarc_library/Discontinuities/Threshold  operator=>=  param_src=Specify via dialog  threshold=0.5  duration=0.1
      settings: SourceProductName=QUARC Targets
  Time : quarc_library/Sources/Time/Time  time_source=Wall clock  sample_time=qc_get_step_size
  Communication Issue (0,1) : Outport  VectorParamsAs1DForOutWhenUnconnected=off
  wires:
  Error/1 -> MATLAB Function/3(error)
  MATLAB Function/1(stream_connection_loss) -> Threshold/1
  State/1 -> MATLAB Function/2(state)
  Time/1 -> MATLAB Function/1(time)
  Threshold/2 -> Terminator2/1
  Data Type Conversion/1 -> Communication Issue (0,1)/1
  Threshold/1 -> Data Type Conversion/1

== system QD2_MissionCtrl_Swarm_6x_R2021a/Communication V3/Detect Communication loss ==
  State : Inport
  Error : Inport  Port=2
  Data Type Conversion : DataTypeConversion
  MATLAB Function : MATLAB Function  TreatAsAtomicUnit=on
  Terminator2 : Terminator
  Threshold : quarc_library/Discontinuities/Threshold  operator=>=  param_src=Specify via dialog  threshold=0.5  duration=0.1
      settings: SourceProductName=QUARC Targets
  Time : quarc_library/Sources/Time/Time  time_source=Wall clock  sample_time=qc_get_step_size
  Communication Issue (0,1) : Outport  VectorParamsAs1DForOutWhenUnconnected=off
  wires:
  Threshold/1 -> Data Type Conversion/1
  Data Type Conversion/1 -> Communication Issue (0,1)/1
  Threshold/2 -> Terminator2/1
  Time/1 -> MATLAB Function/1(time)
  State/1 -> MATLAB Function/2(state)
  MATLAB Function/1(stream_connection_loss) -> Threshold/1
  Error/1 -> MATLAB Function/3(error)

== system QD2_MissionCtrl_Swarm_6x_R2021a/Communication V4/Detect Communication loss ==
  State : Inport
  Error : Inport  Port=2
  Data Type Conversion : DataTypeConversion
  MATLAB Function : MATLAB Function  TreatAsAtomicUnit=on
  Terminator2 : Terminator
  Threshold : quarc_library/Discontinuities/Threshold  operator=>=  param_src=Specify via dialog  threshold=0.5  duration=0.1
      settings: SourceProductName=QUARC Targets
  Time : quarc_library/Sources/Time/Time  time_source=Wall clock  sample_time=qc_get_step_size
  Communication Issue (0,1) : Outport  VectorParamsAs1DForOutWhenUnconnected=off
  wires:
  Error/1 -> MATLAB Function/3(error)
  MATLAB Function/1(stream_connection_loss) -> Threshold/1
  State/1 -> MATLAB Function/2(state)
  Time/1 -> MATLAB Function/1(time)
  Threshold/2 -> Terminator2/1
  Data Type Conversion/1 -> Communication Issue (0,1)/1
  Threshold/1 -> Data Type Conversion/1

== system QD2_MissionCtrl_Swarm_6x_R2021a/Communication V5/Detect Communication loss ==
  State : Inport
  Error : Inport  Port=2
  Data Type Conversion : DataTypeConversion
  MATLAB Function : MATLAB Function  TreatAsAtomicUnit=on
  Terminator2 : Terminator
  Threshold : quarc_library/Discontinuities/Threshold  operator=>=  param_src=Specify via dialog  threshold=0.5  duration=0.1
      settings: SourceProductName=QUARC Targets
  Time : quarc_library/Sources/Time/Time  time_source=Wall clock  sample_time=qc_get_step_size
  Communication Issue (0,1) : Outport  VectorParamsAs1DForOutWhenUnconnected=off
  wires:
  Threshold/1 -> Data Type Conversion/1
  Data Type Conversion/1 -> Communication Issue (0,1)/1
  Threshold/2 -> Terminator2/1
  Time/1 -> MATLAB Function/1(time)
  State/1 -> MATLAB Function/2(state)
  MATLAB Function/1(stream_connection_loss) -> Threshold/1
  Error/1 -> MATLAB Function/3(error)

== system QD2_MissionCtrl_Swarm_6x_R2021a/Communication V6/Detect Communication loss ==
  State : Inport
  Error : Inport  Port=2
  Data Type Conversion : DataTypeConversion
  MATLAB Function : MATLAB Function  TreatAsAtomicUnit=on
  Terminator2 : Terminator
  Threshold : quarc_library/Discontinuities/Threshold  operator=>=  param_src=Specify via dialog  threshold=0.5  duration=0.1
      settings: SourceProductName=QUARC Targets
  Time : quarc_library/Sources/Time/Time  time_source=Wall clock  sample_time=qc_get_step_size
  Communication Issue (0,1) : Outport  VectorParamsAs1DForOutWhenUnconnected=off
  wires:
  Error/1 -> MATLAB Function/3(error)
  MATLAB Function/1(stream_connection_loss) -> Threshold/1
  State/1 -> MATLAB Function/2(state)
  Time/1 -> MATLAB Function/1(time)
  Threshold/2 -> Terminator2/1
  Data Type Conversion/1 -> Communication Issue (0,1)/1
  Threshold/1 -> Data Type Conversion/1

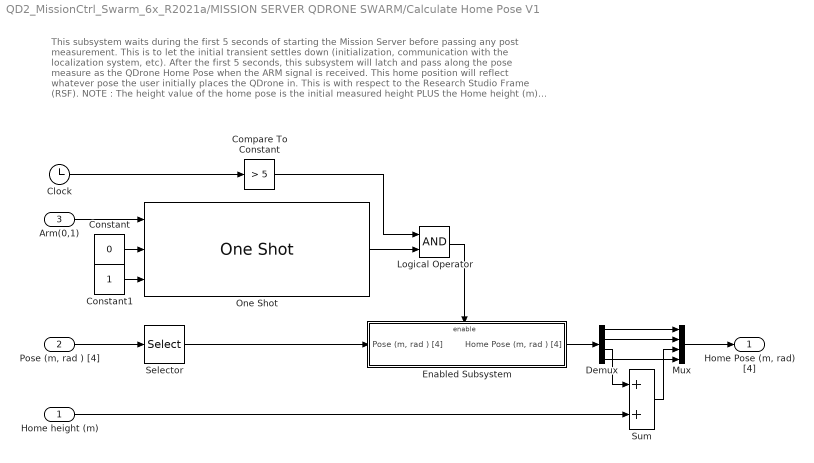
== system QD2_MissionCtrl_Swarm_6x_R2021a/MISSION SERVER QDRONE SWARM/Calculate Home Pose V1 ==
  note: This subsystem waits during the first 5 seconds of starting the Mission Server before passing any post measurement.
      | This is to let the initial transient settles down (initialization, communication with the localization system, etc).
      | After the first 5 seconds, this subsystem will latch and pass along the pose measure as the QDrone Home Pose when
      | the ARM signal is received.
      | This home position will reflect whatever pose the user initially places the QDrone in.
      | This is with respect to the Research Studio Frame (RSF).
      |
      | NOTE : The height value of the home pose is the initial measured height PLUS the Home height (m) input value.
  Home height (m) : Inport
  "Pose (m, rad ) [4]" : Inport  Port=2
  Arm(0,1) : Inport  Port=3
  Clock : Clock
  Compare To Constant : simulink/Logic and Bit Operations/Compare To Constant  relop=>  const=5  OutDataTypeStr=boolean
  Constant : Constant  Value=0
  Constant1 : Constant
  Demux : Demux
  Enabled Subsystem : Subsystem  TreatAsAtomicUnit=on
  Logical Operator : Logic  AllPortsSameDT=off  OutDataTypeStr=boolean
  Mux : Mux
  One Shot : quarc_library/Discontinuities/One Shot  trigger_type=Rising edge  redun_pulse=Ignore extraneous pulse  width_source=Specify via dialog  pulse_width=1/qc_get_step_size
      settings: SourceProductName=QUARC Targets
  Selector : Selector  InputPortWidth=6  IndexOptions=Index vector (dialog)  Indices=[1:3,6]  OutputSizes=1
  Sum : Sum
  "Home Pose (m, rad) [4]" : Outport  VectorParamsAs1DForOutWhenUnconnected=off
  wires:
  Constant/1 -> One Shot/2
  Constant1/1 -> One Shot/3
  Arm(0,1)/1 -> One Shot/1
  One Shot/1 -> Logical Operator/2
  "Pose (m, rad ) [4]"/1 -> Selector/1
  Clock/1 -> Compare To Constant/1
  Compare To Constant/1 -> Logical Operator/1
  Logical Operator/1 -> Enabled Subsystem/Enable
  Enabled Subsystem/1("Home Pose (m, rad ) [4]") -> Demux/1
  Demux/1 -> Mux/1
  Demux/2 -> Mux/2
  Demux/4 -> Mux/4
  Demux/3 -> Sum/1
  Sum/1 -> Mux/3
  Home height (m)/1 -> Sum/2
  Mux/1 -> "Home Pose (m, rad) [4]"/1
  Selector/1 -> Enabled Subsystem/1("Pose (m, rad ) [4] ")

== system QD2_MissionCtrl_Swarm_6x_R2021a/MISSION SERVER QDRONE SWARM/Calculate Home Pose V2 ==
  note: This subsystem waits during the first 5 seconds of starting the Mission Server before passing any post measurement.
      | This is to let the initial transient settles down (initialization, communication with the localization system, etc).
      | After the first 5 seconds, this subsystem will latch and pass along the pose measure as the QDrone Home Pose when
      | the ARM signal is received.
      | This home position will reflect whatever pose the user initially places the QDrone in.
      | This is with respect to the Research Studio Frame (RSF).
      |
      | NOTE : The height value of the home pose is the initial measured height PLUS the Home height (m) input value.
  Home height (m) : Inport
  "Pose (m, rad ) [4]" : Inport  Port=2
  Arm(0,1) : Inport  Port=3
  Clock : Clock
  Compare To Constant : simulink/Logic and Bit Operations/Compare To Constant  relop=>  const=5  OutDataTypeStr=boolean
  Constant : Constant  Value=0
  Constant1 : Constant
  Demux : Demux
  Enabled Subsystem : Subsystem  TreatAsAtomicUnit=on
  Logical Operator : Logic  AllPortsSameDT=off  OutDataTypeStr=boolean
  Mux : Mux
  One Shot : quarc_library/Discontinuities/One Shot  trigger_type=Rising edge  redun_pulse=Ignore extraneous pulse  width_source=Specify via dialog  pulse_width=1/qc_get_step_size
      settings: SourceProductName=QUARC Targets
  Selector : Selector  InputPortWidth=6  IndexOptions=Index vector (dialog)  Indices=[1:3,6]  OutputSizes=1
  Sum : Sum
  "Home Pose (m, rad) [4]" : Outport  VectorParamsAs1DForOutWhenUnconnected=off
  wires:
  Constant/1 -> One Shot/2
  Constant1/1 -> One Shot/3
  Arm(0,1)/1 -> One Shot/1
  One Shot/1 -> Logical Operator/2
  "Pose (m, rad ) [4]"/1 -> Selector/1
  Clock/1 -> Compare To Constant/1
  Compare To Constant/1 -> Logical Operator/1
  Logical Operator/1 -> Enabled Subsystem/Enable
  Enabled Subsystem/1("Home Pose (m, rad ) [4]") -> Demux/1
  Demux/1 -> Mux/1
  Demux/2 -> Mux/2
  Demux/4 -> Mux/4
  Demux/3 -> Sum/1
  Sum/1 -> Mux/3
  Home height (m)/1 -> Sum/2
  Mux/1 -> "Home Pose (m, rad) [4]"/1
  Selector/1 -> Enabled Subsystem/1("Pose (m, rad ) [4] ")

== system QD2_MissionCtrl_Swarm_6x_R2021a/MISSION SERVER QDRONE SWARM/Calculate Home Pose V3 ==
  note: This subsystem waits during the first 5 seconds of starting the Mission Server before passing any post measurement.
      | This is to let the initial transient settles down (initialization, communication with the localization system, etc).
      | After the first 5 seconds, this subsystem will latch and pass along the pose measure as the QDrone Home Pose when
      | the ARM signal is received.
      | This home position will reflect whatever pose the user initially places the QDrone in.
      | This is with respect to the Research Studio Frame (RSF).
      |
      | NOTE : The height value of the home pose is the initial measured height PLUS the Home height (m) input value.
  Home height (m) : Inport
  "Pose (m, rad ) [4]" : Inport  Port=2
  Arm(0,1) : Inport  Port=3
  Clock : Clock
  Compare To Constant : simulink/Logic and Bit Operations/Compare To Constant  relop=>  const=5  OutDataTypeStr=boolean
  Constant : Constant  Value=0
  Constant1 : Constant
  Demux : Demux
  Enabled Subsystem : Subsystem  TreatAsAtomicUnit=on
  Logical Operator : Logic  AllPortsSameDT=off  OutDataTypeStr=boolean
  Mux : Mux
  One Shot : quarc_library/Discontinuities/One Shot  trigger_type=Rising edge  redun_pulse=Ignore extraneous pulse  width_source=Specify via dialog  pulse_width=1/qc_get_step_size
      settings: SourceProductName=QUARC Targets
  Selector : Selector  InputPortWidth=6  IndexOptions=Index vector (dialog)  Indices=[1:3,6]  OutputSizes=1
  Sum : Sum
  "Home Pose (m, rad) [4]" : Outport  VectorParamsAs1DForOutWhenUnconnected=off
  wires:
  Constant/1 -> One Shot/2
  Constant1/1 -> One Shot/3
  Arm(0,1)/1 -> One Shot/1
  One Shot/1 -> Logical Operator/2
  "Pose (m, rad ) [4]"/1 -> Selector/1
  Clock/1 -> Compare To Constant/1
  Compare To Constant/1 -> Logical Operator/1
  Logical Operator/1 -> Enabled Subsystem/Enable
  Enabled Subsystem/1("Home Pose (m, rad ) [4]") -> Demux/1
  Demux/1 -> Mux/1
  Demux/2 -> Mux/2
  Demux/4 -> Mux/4
  Demux/3 -> Sum/1
  Sum/1 -> Mux/3
  Home height (m)/1 -> Sum/2
  Mux/1 -> "Home Pose (m, rad) [4]"/1
  Selector/1 -> Enabled Subsystem/1("Pose (m, rad ) [4] ")
